simulink model "Equation_Bicycle_Model"  (R2022a)
settings: Solver=VariableStepAuto  StartTime=0.0  StopTime=10.0  RelTol=1e-3
settings Model: Creator=Joakim Nylander N  LastModifiedBy=Joakim Nylander N

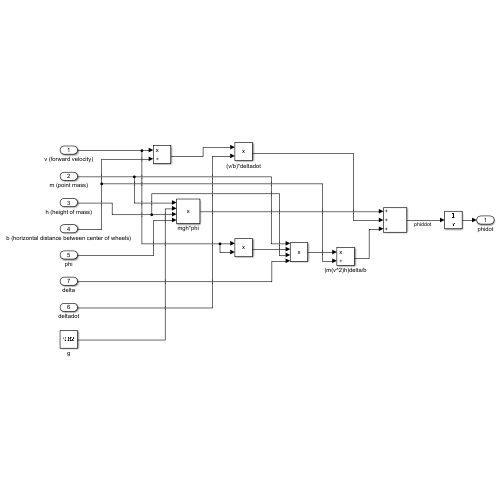
[thumbnail: Simulink's stored preview of the top-level diagram]
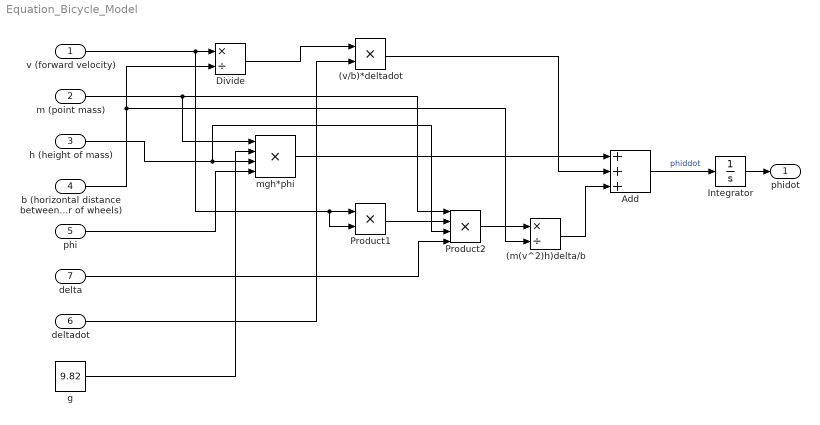
== system Equation_Bicycle_Model ==
  v (forward velocity) : Inport
  m (point mass) : Inport  Port=2
  h (height of mass) : Inport  Port=3
  b (horizontal distance between center of wheels) : Inport  Port=4
  phi : Inport  Port=5
  deltadot : Inport  Port=6
  delta : Inport  Port=7
  (m(v^2)h)delta/b : Product  Inputs=*/
  (v/b)*deltadot : Product
  Add : Sum  Inputs=+++
  Divide : Product  Inputs=*/
  Integrator : Integrator
  Product1 : Product
  Product2 : Product  Inputs=4
  g : Constant  Value=9.82
  mgh*phi : Product  Inputs=4
  phidot : Outport
  wires:
  g/1 -> mgh*phi/2
  m (point mass)/1 -> Product2/1, mgh*phi/1
  h (height of mass)/1 -> Product2/3, mgh*phi/3
  phi/1 -> mgh*phi/4
  v (forward velocity)/1 -> Product1/2, Product1/1, Divide/1
  b (horizontal distance between center of wheels)/1 -> (m(v^2)h)delta/b/2, Divide/2
  Divide/1 -> (v/b)*deltadot/1
  deltadot/1 -> (v/b)*deltadot/2
  mgh*phi/1 -> Add/1
  (v/b)*deltadot/1 -> Add/2
  Product1/1 -> Product2/2
  delta/1 -> Product2/4
  Product2/1 -> (m(v^2)h)delta/b/1
  (m(v^2)h)delta/b/1 -> Add/3
  Add/1 -> Integrator/1  "phiddot"
  Integrator/1 -> phidot/1
